simulink model "first_order_ramp"  (R2023b)
settings: Solver=VariableStepAuto  StartTime=0.0  StopTime=10.0  RelTol=1e-3
libraries: simulink x1
settings Model: Creator=Maxwe  LastModifiedBy=Maxwe
settings HardwareCC: ProdHWDeviceType=AMD->x86-64 (Windows64)

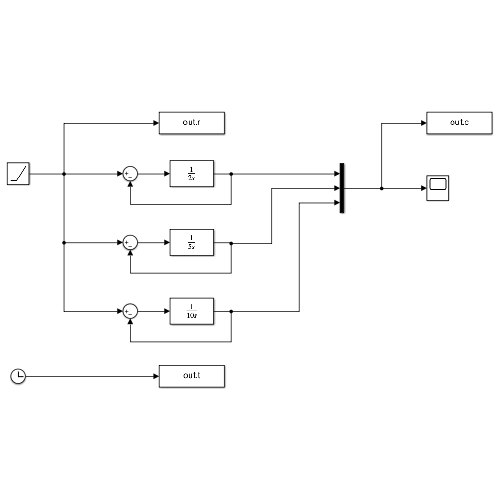
[thumbnail: Simulink's stored preview of the top-level diagram]
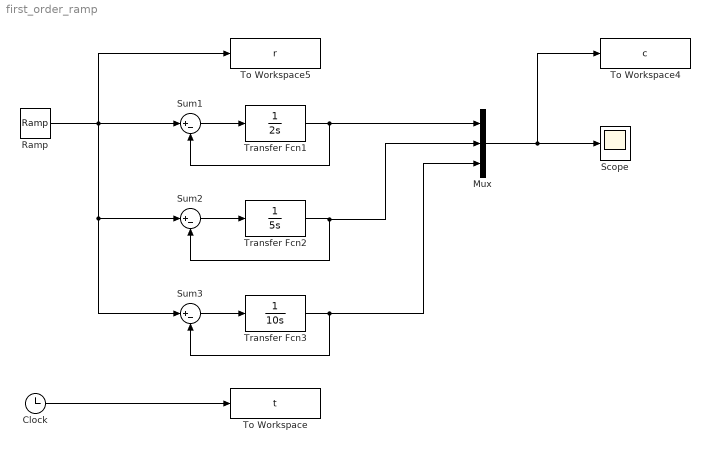
== system first_order_ramp ==
  Clock : Clock
  Mux : Mux  Inputs=3
  Ramp : simulink/Sources/Ramp  slope=1  start=0  InitialOutput=0
  Scope : Scope
  Sum1 : Sum  Inputs=|+-
  Sum2 : Sum  Inputs=|+-
  Sum3 : Sum  Inputs=|+-
  To Workspace : ToWorkspace  VariableName=t  SampleTime=-1
      settings: Save2DSignal=2-D array (concatenate along first dimension)
  To Workspace4 : ToWorkspace  VariableName=c  SampleTime=-1
      settings: Save2DSignal=2-D array (concatenate along first dimension)
  To Workspace5 : ToWorkspace  VariableName=r  SampleTime=-1
      settings: Save2DSignal=2-D array (concatenate along first dimension)
  Transfer Fcn1 : TransferFcn  Denominator=[2 0]
  Transfer Fcn2 : TransferFcn  Denominator=[5 0]
  Transfer Fcn3 : TransferFcn  Denominator=[10 0]
  wires:
  Clock/1 -> To Workspace/1
  Mux/1 -> To Workspace4/1, Scope/1
  Ramp/1 -> Sum3/1, Sum2/1, Sum1/1, To Workspace5/1
  Sum1/1 -> Transfer Fcn1/1
  Sum2/1 -> Transfer Fcn2/1
  Transfer Fcn1/1 -> Mux/1, Sum1/2
  Transfer Fcn2/1 -> Mux/2, Sum2/2
  Sum3/1 -> Transfer Fcn3/1
  Transfer Fcn3/1 -> Mux/3, Sum3/2
